simulink model "Loss_Test_circuit_fromDataSheet"  (R2016a)
settings: Solver=FixedStepAuto  StartTime=0.0  StopTime=10.0  FixedStep=0.0001  RelTol=1e-3
undefined symbols (not defined in the file or in its folder): fsw, Lp, Rg_off, Rg_on, td_off, td_on, tr
libraries: elec_lib x16, fl_lib x7, nesl_utility x7
settings Model: Creator=syf  LastModifiedBy=syf

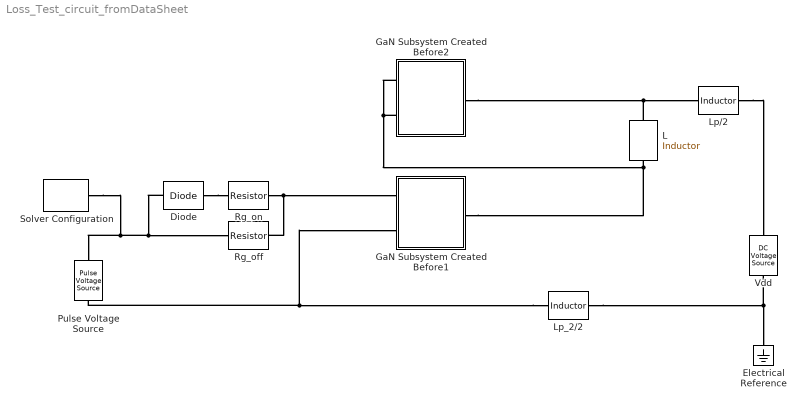
== system Loss_Test_circuit_fromDataSheet ==
  Diode : elec_lib/Semiconductor Devices/Diode  ModelType=1  Vf=0.6 V  Ron=0.3 Ohm  Goff=1e-8 S  Rz=0.3 Ohm  Vz=50 V  C_PWL=5 pF  prmExp=1  I12=[ 0.0137 0.545 ] A  V12=[ 0.6 0.7 ] V  I1=0.0137 A  V1=0.6 V  RS=0.01 Ohm  IS=1e-12 A  Tmeas=25 degC  ec=1  BV=Inf V  C_param=1  CJ0=5 pF  VJ=1 V  Mgrad=0.5  Vvec=[ 0.1 10 100 ] V  Cvec=[ 3.5 1 0.4 ] pF  FC=0.5  Q_param=1  Irrm=-7.15 A  iF=4 A  didt=-750 A/us  trr=115 ns  TT=50 ns  tau=100 ns  T_param=1  IS_T2=1.25e-7 A  I1_T2=0.245 A  V1_T2=0.5 V  Tmeas2=125 degC  EG_param=1  EG=1.11 eV  XTI_param=1  XTI=3  dBVdT=0 V/K  Tdevice=25 degC  Rth=[ 0 10 ] K/W  thermal_mass_parameterization=1  thermal_mass=[ 0 1 ] J/K  thermal_time_constant=[ 0 10 ] s  thermal_mass_initial_temperatures=[ 25 25 ] degC
  Electrical Reference : fl_lib/Electrical/Electrical Elements/Electrical Reference
  GaN Subsystem Created Before1 : Subsystem
  GaN Subsystem Created Before2 : Subsystem
  L : elec_lib/Passive Devices/Inductor  l=L H  L_tol=20  enable_L_tol=0  tol_distribution=1  nSigma=4  r=0 Ohm  g=1e-9 1/Ohm  initI=0 A  enable_operating_limits=0  operating_limit_action=2  max_working_current=1 A  power_rating=1 W  enable_faults=0  fault_action=1  lambdaPercent=50  k_faulted=0.9999 Ohm  turnsShort=0  openCct=0  groundShort=0  groundShortG=0 1/Ohm  tau_fault=0.001 s  enable_temporal_fault=0  t_fault=1 s  enable_behavioral_fault=0  max_permissible_voltage=100 V  n_fail_on_voltage=1  max_permissible_current=1 A  t_fail_on_current=1 s
  Lp/2 : elec_lib/Passive Devices/Inductor  l=Lp/2 H  L_tol=20  enable_L_tol=0  tol_distribution=1  nSigma=4  r=0 Ohm  g=1e-9 1/Ohm  initI=0 A  enable_operating_limits=0  operating_limit_action=2  max_working_current=1 A  power_rating=1 W  enable_faults=0  fault_action=1  lambdaPercent=50  k_faulted=0.9999 Ohm  turnsShort=0  openCct=0  groundShort=0  groundShortG=0 1/Ohm  tau_fault=0.001 s  enable_temporal_fault=0  t_fault=1 s  enable_behavioral_fault=0  max_permissible_voltage=100 V  n_fail_on_voltage=1  max_permissible_current=1 A  t_fail_on_current=1 s
  Lp_2/2 : elec_lib/Passive Devices/Inductor  l=Lp/2 H  L_tol=20  enable_L_tol=0  tol_distribution=1  nSigma=4  r=0 Ohm  g=1e-9 1/Ohm  initI=0 A  enable_operating_limits=0  operating_limit_action=2  max_working_current=1 A  power_rating=1 W  enable_faults=0  fault_action=1  lambdaPercent=50  k_faulted=0.9999 Ohm  turnsShort=0  openCct=0  groundShort=0  groundShortG=0 1/Ohm  tau_fault=0.001 s  enable_temporal_fault=0  t_fault=1 s  enable_behavioral_fault=0  max_permissible_voltage=100 V  n_fail_on_voltage=1  max_permissible_current=1 A  t_fail_on_current=1 s
  Pulse Voltage Source : elec_lib/Additional Components/SPICE-Compatible Components/Sources/Pulse Voltage Source  V1=0 V  V2=6 V  TD=0 s  TR=tr+td_on s  TF=tf+td_off s  PW=0.5/fsw s  PER=1/fsw s
  Rg_off : elec_lib/Passive Devices/Resistor  R=Rg_off Ohm  R_tol=5  enable_R_tol=0  tol_distribution=1  nSigma=4  enable_operating_limits=0  operating_limit_action=2  max_working_voltage=100 V  power_rating=1 W  enable_faults=0  fault_action=1  R_faulted=Inf Ohm  enable_temporal_fault=0  t_fault=1 s  enable_behavioral_fault=0  max_permissible_current=1 A  t_fail_on_current=1 s  noise_mode=0  sample_time=0.001 s  repeatability=1  auto_seed=3213286623  user_seed=0  Tdevice=25 degC  alpha=0.00393 1/K  Tmeas=25 degC  thermal_mass=100 J/K  initial_temperature=25 degC  power_derating_T1=70 degC  power_derating_T2=155 degC  operating_temperature_range_vec=[ -50 150 ] degC
  Rg_on : elec_lib/Passive Devices/Resistor  R=Rg_on Ohm  R_tol=5  enable_R_tol=0  tol_distribution=1  nSigma=4  enable_operating_limits=0  operating_limit_action=2  max_working_voltage=100 V  power_rating=1 W  enable_faults=0  fault_action=1  R_faulted=Inf Ohm  enable_temporal_fault=0  t_fault=1 s  enable_behavioral_fault=0  max_permissible_current=1 A  t_fail_on_current=1 s  noise_mode=0  sample_time=0.001 s  repeatability=1  auto_seed=2787929736  user_seed=0  Tdevice=25 degC  alpha=0.00393 1/K  Tmeas=25 degC  thermal_mass=100 J/K  initial_temperature=25 degC  power_derating_T1=70 degC  power_derating_T2=155 degC  operating_temperature_range_vec=[ -50 150 ] degC
  Solver Configuration : nesl_utility/Solver Configuration  PhysicalDomain=network_engine_domain  SubClassName=solver  LeftPortType=input  RightPortType=generic  Accelerate=off  Tones=[]  Harmonics=[]  SimulateNoise=off  Profile=off  UseLocalSampling=off  EnableSwitchedLinearOptims=on  FrequencyDomain=off  UseCCode=off  RelTol=0.001  AbsTol=1e-06  MinStep=1e-09  ToWorkspace=off  RevertToSquareIcSolve=off  NumHomotopyIterations=100  PhasorMode=off  PhasorModeNumHarmonics=1  OverrideAbsTol=off  DoDC=off  ResidualTolerance=1e-09  UseLocalSolver=off  LocalSolverChoice=NE_BACKWARD_EULER_ADVANCER  LocalSolverSampleTime=0.001  DoFixedCost=off  MaxNonlinIter=3  MaxModeIter=2  LinearAlgebra=Sparse  DelaysMemoryBudget=1024  AutomaticFiltering=on  FilteringTimeConstant=0.001
  Vdd : elec_lib/Additional Components/SPICE-Compatible Components/Sources/DC Voltage Source  DC=Vds V
  connections:
  Lp/2/RConn1 -- Vdd/LConn1
  Lp_2/2/RConn1 -- Electrical Reference/LConn1 -- Vdd/RConn1
  Diode/RConn1 -- Rg_on/LConn1
  Diode/LConn1 -- Solver Configuration/RConn1 -- Pulse Voltage Source/LConn1 -- Rg_off/LConn1
  L/LConn1 -- Lp/2/LConn1 -- GaN Subsystem Created Before2/RConn1
  GaN Subsystem Created Before1/RConn1 -- GaN Subsystem Created Before2/LConn1 -- GaN Subsystem Created Before2/LConn2 -- L/RConn1
  Rg_on/RConn1 -- Rg_off/RConn1 -- GaN Subsystem Created Before1/LConn1
  Lp_2/2/LConn1 -- Pulse Voltage Source/RConn1 -- GaN Subsystem Created Before1/LConn2

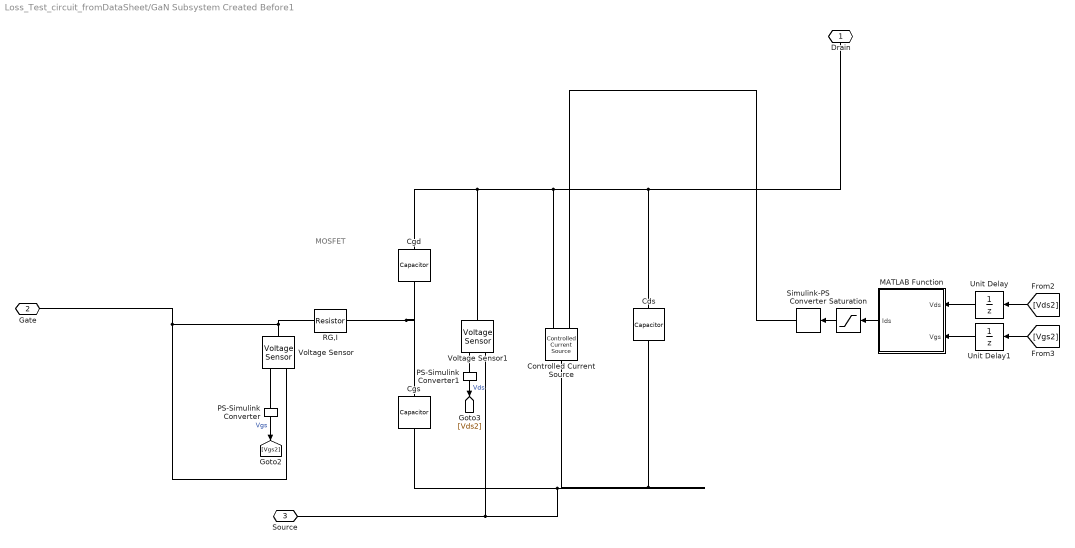
== system Loss_Test_circuit_fromDataSheet/GaN Subsystem Created Before1 ==
  note: MOSFET
  Cds : elec_lib/Passive Devices/Capacitor  enable_table=0  c=63 pF  Cvec=[ 1e-5 1e-6 ] F  Vvec=[ 0 10 ] V  CV_table_symmetry=1  C_tol=5  enable_C_tol=0  tol_distribution=1  nSigma=4  r=1e-6 Ohm  g=0 1/Ohm  initV=0 V  enable_operating_limits=0  operating_limit_action=2  max_working_voltage_range=[ -25 25 ] V  power_rating=1 W  enable_faults=0  fault_action=1  Cscale_faulted=100  R_faulted=0.001 Ohm  G_faulted=0 1/Ohm  tau_fault=0.001 s  enable_temporal_fault=0  t_fault=1 s  enable_behavioral_fault=0  max_permissible_voltage_range=[ -100 100 ] V  t_fail_on_voltage=1 s
  Cgd : elec_lib/Passive Devices/Capacitor  enable_table=0  c=2 pF  Cvec=[ 1e-5 1e-6 ] F  Vvec=[ 0 10 ] V  CV_table_symmetry=1  C_tol=5  enable_C_tol=0  tol_distribution=1  nSigma=4  r=1e-6 Ohm  g=0 1/Ohm  initV=0 V  enable_operating_limits=0  operating_limit_action=2  max_working_voltage_range=[ -25 25 ] V  power_rating=1 W  enable_faults=0  fault_action=1  Cscale_faulted=100  R_faulted=0.001 Ohm  G_faulted=0 1/Ohm  tau_fault=0.001 s  enable_temporal_fault=0  t_fault=1 s  enable_behavioral_fault=0  max_permissible_voltage_range=[ -100 100 ] V  t_fail_on_voltage=1 s
  Cgs : elec_lib/Passive Devices/Capacitor  enable_table=0  c=258 pF  Cvec=[ 1e-5 1e-6 ] F  Vvec=[ 0 10 ] V  CV_table_symmetry=1  C_tol=5  enable_C_tol=0  tol_distribution=1  nSigma=4  r=1e-6 Ohm  g=0 1/Ohm  initV=0 V  enable_operating_limits=0  operating_limit_action=2  max_working_voltage_range=[ -25 25 ] V  power_rating=1 W  enable_faults=0  fault_action=1  Cscale_faulted=100  R_faulted=0.001 Ohm  G_faulted=0 1/Ohm  tau_fault=0.001 s  enable_temporal_fault=0  t_fault=1 s  enable_behavioral_fault=0  max_permissible_voltage_range=[ -100 100 ] V  t_fail_on_voltage=1 s
  Controlled Current Source : fl_lib/Electrical/Electrical Sources/Controlled Current Source
  MATLAB Function : MATLAB Function  TreatAsAtomicUnit=on
  PS-Simulink Converter : nesl_utility/PS-Simulink Converter  PhysicalDomain=network_engine_domain  SubClassName=ps_output  LeftPortType=input  RightPortType=output  PseudoPeriodic=off  Frequencies=[]  Unit=1  AffineConversion=off
  PS-Simulink Converter1 : nesl_utility/PS-Simulink Converter  PhysicalDomain=network_engine_domain  SubClassName=ps_output  LeftPortType=input  RightPortType=output  PseudoPeriodic=off  Frequencies=[]  Unit=1  AffineConversion=off
  RG,I : elec_lib/Passive Devices/Resistor  R=1 Ohm  R_tol=5  enable_R_tol=0  tol_distribution=1  nSigma=4  enable_operating_limits=0  operating_limit_action=2  max_working_voltage=100 V  power_rating=1 W  enable_faults=0  fault_action=1  R_faulted=Inf Ohm  enable_temporal_fault=0  t_fault=1 s  enable_behavioral_fault=0  max_permissible_current=1 A  t_fail_on_current=1 s  noise_mode=0  sample_time=0.001 s  repeatability=1  auto_seed=735241226  user_seed=0  Tdevice=25 degC  alpha=0.00393 1/K  Tmeas=25 degC  thermal_mass=100 J/K  initial_temperature=25 degC  power_derating_T1=70 degC  power_derating_T2=155 degC  operating_temperature_range_vec=[ -50 150 ] degC
  Saturation : Saturate  UpperLimit=30  LowerLimit=-30
  Simulink-PS Converter : nesl_utility/Simulink-PS Converter  PhysicalDomain=network_engine_domain  SubClassName=ps_input  LeftPortType=input  RightPortType=output  PseudoPeriodic=off  Frequencies=[]  NoiseDistribution=none  NoiseParameters=[]  Unit=1  AffineConversion=off  InputFiltering=off  SimscapeFilterOrder=1  InputFilterTimeConstant=0.001  UdotUserProvided=1
  Unit Delay : UnitDelay  SampleTime=-1
  Unit Delay1 : UnitDelay  SampleTime=-1
  Voltage Sensor : fl_lib/Electrical/Electrical Sensors/Voltage Sensor
  Voltage Sensor1 : fl_lib/Electrical/Electrical Sensors/Voltage Sensor
  Drain : PMIOPort  Port=1  Side=Right
  Gate : PMIOPort  Port=2  Side=Left
  Source : PMIOPort  Port=3  Side=Left
  wires:
  Unit Delay1/1 -> MATLAB Function/2(Vgs)
  MATLAB Function/1(Ids) -> Saturation/1
  [Vds2] -> Unit Delay/1
  [Vgs2] -> Unit Delay1/1
  Unit Delay/1 -> MATLAB Function/1(Vds)
  Saturation/1 -> Simulink-PS Converter/1
  PS-Simulink Converter1/1 -> [Vds2]  "Vds"
  PS-Simulink Converter/1 -> [Vgs2]  "Vgs"
  connections:
  PS-Simulink Converter1/LConn1 -- Voltage Sensor1/RConn1
  Cgs/LConn1 -- RG,I/RConn1 -- Cgd/RConn1
  Simulink-PS Converter/RConn1 -- Controlled Current Source/RConn1
  Voltage Sensor/RConn1 -- PS-Simulink Converter/LConn1
  Cds/LConn1 -- Drain/RConn1 -- Controlled Current Source/RConn2 -- Voltage Sensor1/LConn1 -- Cgd/LConn1
  Cgs/RConn1 -- Controlled Current Source/LConn1 -- Cds/RConn1 -- Source/RConn1 -- Voltage Sensor1/RConn2
  Voltage Sensor/LConn1 -- Gate/RConn1 -- Voltage Sensor/RConn2 -- RG,I/LConn1

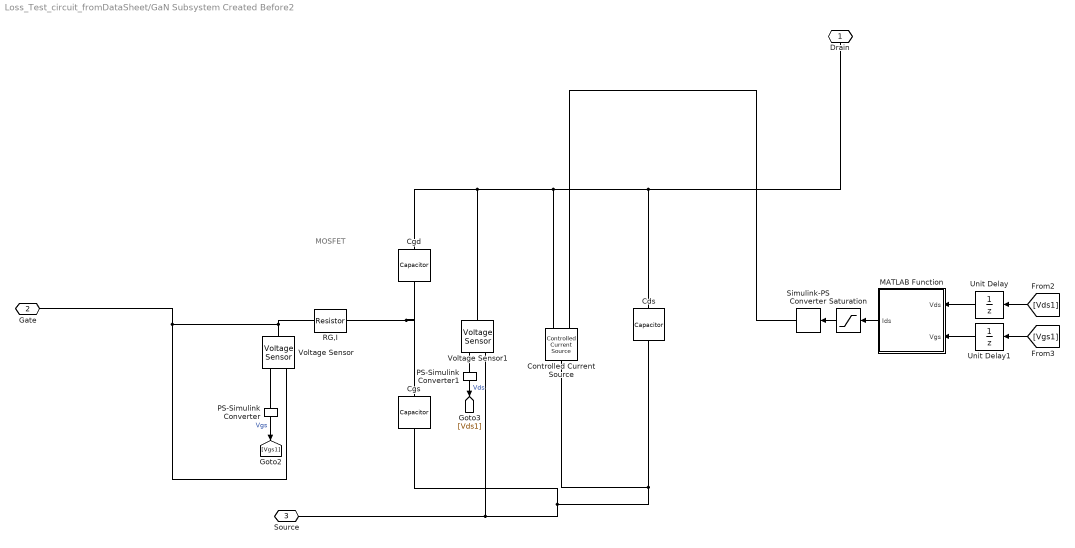
== system Loss_Test_circuit_fromDataSheet/GaN Subsystem Created Before2 ==
  note: MOSFET
  Cds : elec_lib/Passive Devices/Capacitor  enable_table=0  c=63 pF  Cvec=[ 1e-5 1e-6 ] F  Vvec=[ 0 10 ] V  CV_table_symmetry=1  C_tol=5  enable_C_tol=0  tol_distribution=1  nSigma=4  r=1e-6 Ohm  g=0 1/Ohm  initV=0 V  enable_operating_limits=0  operating_limit_action=2  max_working_voltage_range=[ -25 25 ] V  power_rating=1 W  enable_faults=0  fault_action=1  Cscale_faulted=100  R_faulted=0.001 Ohm  G_faulted=0 1/Ohm  tau_fault=0.001 s  enable_temporal_fault=0  t_fault=1 s  enable_behavioral_fault=0  max_permissible_voltage_range=[ -100 100 ] V  t_fail_on_voltage=1 s
  Cgd : elec_lib/Passive Devices/Capacitor  enable_table=0  c=2 pF  Cvec=[ 1e-5 1e-6 ] F  Vvec=[ 0 10 ] V  CV_table_symmetry=1  C_tol=5  enable_C_tol=0  tol_distribution=1  nSigma=4  r=1e-6 Ohm  g=0 1/Ohm  initV=0 V  enable_operating_limits=0  operating_limit_action=2  max_working_voltage_range=[ -25 25 ] V  power_rating=1 W  enable_faults=0  fault_action=1  Cscale_faulted=100  R_faulted=0.001 Ohm  G_faulted=0 1/Ohm  tau_fault=0.001 s  enable_temporal_fault=0  t_fault=1 s  enable_behavioral_fault=0  max_permissible_voltage_range=[ -100 100 ] V  t_fail_on_voltage=1 s
  Cgs : elec_lib/Passive Devices/Capacitor  enable_table=0  c=258 pF  Cvec=[ 1e-5 1e-6 ] F  Vvec=[ 0 10 ] V  CV_table_symmetry=1  C_tol=5  enable_C_tol=0  tol_distribution=1  nSigma=4  r=1e-6 Ohm  g=0 1/Ohm  initV=0 V  enable_operating_limits=0  operating_limit_action=2  max_working_voltage_range=[ -25 25 ] V  power_rating=1 W  enable_faults=0  fault_action=1  Cscale_faulted=100  R_faulted=0.001 Ohm  G_faulted=0 1/Ohm  tau_fault=0.001 s  enable_temporal_fault=0  t_fault=1 s  enable_behavioral_fault=0  max_permissible_voltage_range=[ -100 100 ] V  t_fail_on_voltage=1 s
  Controlled Current Source : fl_lib/Electrical/Electrical Sources/Controlled Current Source
  MATLAB Function : MATLAB Function  TreatAsAtomicUnit=on
  PS-Simulink Converter : nesl_utility/PS-Simulink Converter  PhysicalDomain=network_engine_domain  SubClassName=ps_output  LeftPortType=input  RightPortType=output  PseudoPeriodic=off  Frequencies=[]  Unit=1  AffineConversion=off
  PS-Simulink Converter1 : nesl_utility/PS-Simulink Converter  PhysicalDomain=network_engine_domain  SubClassName=ps_output  LeftPortType=input  RightPortType=output  PseudoPeriodic=off  Frequencies=[]  Unit=1  AffineConversion=off
  RG,I : elec_lib/Passive Devices/Resistor  R=1 Ohm  R_tol=5  enable_R_tol=0  tol_distribution=1  nSigma=4  enable_operating_limits=0  operating_limit_action=2  max_working_voltage=100 V  power_rating=1 W  enable_faults=0  fault_action=1  R_faulted=Inf Ohm  enable_temporal_fault=0  t_fault=1 s  enable_behavioral_fault=0  max_permissible_current=1 A  t_fail_on_current=1 s  noise_mode=0  sample_time=0.001 s  repeatability=1  auto_seed=775743626  user_seed=0  Tdevice=25 degC  alpha=0.00393 1/K  Tmeas=25 degC  thermal_mass=100 J/K  initial_temperature=25 degC  power_derating_T1=70 degC  power_derating_T2=155 degC  operating_temperature_range_vec=[ -50 150 ] degC
  Saturation : Saturate  UpperLimit=30  LowerLimit=-30
  Simulink-PS Converter : nesl_utility/Simulink-PS Converter  PhysicalDomain=network_engine_domain  SubClassName=ps_input  LeftPortType=input  RightPortType=output  PseudoPeriodic=off  Frequencies=[]  NoiseDistribution=none  NoiseParameters=[]  Unit=1  AffineConversion=off  InputFiltering=off  SimscapeFilterOrder=1  InputFilterTimeConstant=0.001  UdotUserProvided=1
  Unit Delay : UnitDelay  SampleTime=-1
  Unit Delay1 : UnitDelay  SampleTime=-1
  Voltage Sensor : fl_lib/Electrical/Electrical Sensors/Voltage Sensor
  Voltage Sensor1 : fl_lib/Electrical/Electrical Sensors/Voltage Sensor
  Drain : PMIOPort  Port=1  Side=Right
  Gate : PMIOPort  Port=2  Side=Left
  Source : PMIOPort  Port=3  Side=Left
  wires:
  PS-Simulink Converter/1 -> [Vgs1]  "Vgs"
  PS-Simulink Converter1/1 -> [Vds1]  "Vds"
  Saturation/1 -> Simulink-PS Converter/1
  Unit Delay/1 -> MATLAB Function/1(Vds)
  [Vgs1] -> Unit Delay1/1
  [Vds1] -> Unit Delay/1
  MATLAB Function/1(Ids) -> Saturation/1
  Unit Delay1/1 -> MATLAB Function/2(Vgs)
  connections:
  Gate/RConn1 -- Voltage Sensor/RConn2 -- RG,I/LConn1 -- Voltage Sensor/LConn1
  Source/RConn1 -- Voltage Sensor1/RConn2 -- Cgs/RConn1 -- Cds/RConn1 -- Controlled Current Source/LConn1
  Drain/RConn1 -- Cds/LConn1 -- Cgd/LConn1 -- Voltage Sensor1/LConn1 -- Controlled Current Source/RConn2
  Voltage Sensor/RConn1 -- PS-Simulink Converter/LConn1
  Simulink-PS Converter/RConn1 -- Controlled Current Source/RConn1
  Cgd/RConn1 -- Cgs/LConn1 -- RG,I/RConn1
  PS-Simulink Converter1/LConn1 -- Voltage Sensor1/RConn1

== matlab function Loss_Test_circuit_fromDataSheet/GaN Subsystem Created Before1/MATLAB Function ==
  data: Vds input; Ids output; Vgs input
function Ids = fcn(Vds, Vgs)
% b1=2.035;
% c1=0.124;
% d1=1.159;
% e1=-0.204;
% b2=2.054;
% c2=0.153;
% m1=30.972;
% n1=-4.48;
% l1=4.316e-3;
% l2=-1.091e-3;
% h1=3.771e-3;
% h2=-7.872e-3;
% T=25;
% k1=0.283;
% k2=7.114;
% Vgd=Vgs-Vds;

% K1_T=k1*(1-l1*(T-25));
% K2_T=k2*(1-l2*(T-25));
% P1_T=(1-h1*(T-25));
% P2_T=(1-h2*(T-25));
% 
% if Vds>0
%     Ids=  K1_T*log(1+exp((Vgs-b1)/c1))*(((m1+n1*Vgs)*Vds)/(1+P1_T*(d1+e1*Vgs)*Vds));
% else
%     Ids= K2_T*log(1+exp((Vgd-b2)/c2))*(Vds/(1-P2_T*Vds));

cur=0.85/3.6*0.069*75/80*295;
x0=0.31;
x1=0.255;
T=25;

        if Vds==0
            Vds=0.001;
        end
        if Vds>0
            Ids=cur*(0.8*((T-25+273)/300)^-2.7)*log(1+exp(26*(Vgs-7.9+6.2)))*Vds/(1+max((x0+x1*(Vgs+4.1)),0.2)*Vds);
        else
            Ids=-cur*(0.8*((T-25+273)/300)^-2.7)*log(1+exp(21*((Vgs-Vds)-7.9+6.2)))*(-Vds)/(1+max((x0+x1*((Vgs-Vds)+6.1)),0.2)*(-Vds));
        end
end

== matlab function Loss_Test_circuit_fromDataSheet/GaN Subsystem Created Before2/MATLAB Function ==
  data: Vds input; Ids output; Vgs input
function Ids = fcn(Vds, Vgs)
% b1=2.035;
% c1=0.124;
% d1=1.159;
% e1=-0.204;
% b2=2.054;
% c2=0.153;
% m1=30.972;
% n1=-4.48;
% l1=4.316e-3;
% l2=-1.091e-3;
% h1=3.771e-3;
% h2=-7.872e-3;
% T=25;
% k1=0.283;
% k2=7.114;
% Vgd=Vgs-Vds;

% K1_T=k1*(1-l1*(T-25));
% K2_T=k2*(1-l2*(T-25));
% P1_T=(1-h1*(T-25));
% P2_T=(1-h2*(T-25));
% 
% if Vds>0
%     Ids=  K1_T*log(1+exp((Vgs-b1)/c1))*(((m1+n1*Vgs)*Vds)/(1+P1_T*(d1+e1*Vgs)*Vds));
% else
%     Ids= K2_T*log(1+exp((Vgd-b2)/c2))*(Vds/(1-P2_T*Vds));

cur=0.85/3.6*0.069*75/80*295;
x0=0.31;
x1=0.255;
T=25;

        if Vds==0
            Vds=0.001;
        end
        if Vds>0
            Ids=cur*(0.8*((T-25+273)/300)^-2.7)*log(1+exp(26*(Vgs-7.9+6.2)))*Vds/(1+max((x0+x1*(Vgs+4.1)),0.2)*Vds);
        else
            Ids=-cur*(0.8*((T-25+273)/300)^-2.7)*log(1+exp(21*((Vgs-Vds)-7.9+6.2)))*(-Vds)/(1+max((x0+x1*((Vgs-Vds)+6.1)),0.2)*(-Vds));
        end
end
